simulink model "three_and_5_pole_jojo"  (R2025b)
settings: Solver=VariableStepAuto  StartTime=0.0  StopTime=20  RelTol=1e-3
model workspace (MAT data in the model file):
  Ki = 1546
  Kp = 7142.9
  Var = 0
  b = 50
  m = 1000
  u = 10
settings Model: Creator=clee1  LastModifiedBy=coven
settings SolverCC: AlgebraicLoopSolver=TrustRegion
settings DebuggingCC: UnconnectedInputMsg=warning  UnconnectedOutputMsg=warning  UnconnectedLineMsg=warning
settings ModelReferenceCC: EnableRefExpFcnMdlSchedulingChecks=on
settings RTWCC: GPUComputeCapability=3.5

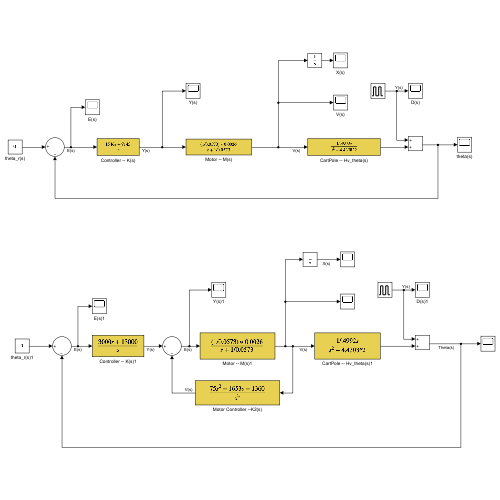
[thumbnail: Simulink's stored preview of the top-level diagram]
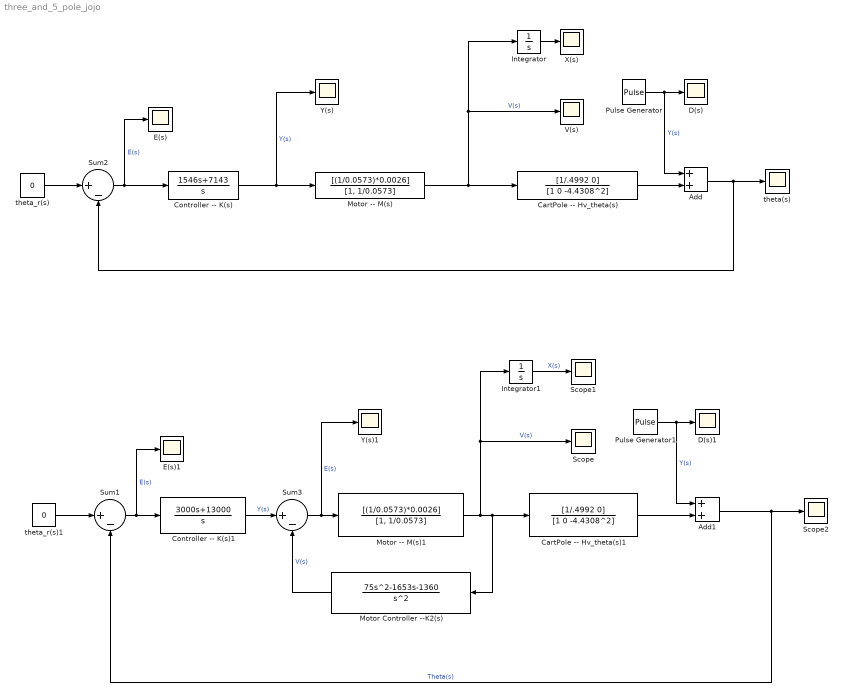
== system three_and_5_pole_jojo ==
  Add : Sum
  Add1 : Sum
  "CartPole -- Hv_theta(s)" : TransferFcn  Numerator=[1/.4992 0]  Denominator=[1 0 -4.4308^2]  ContinuousStateAttributes="\"Controller\""
  "CartPole -- Hv_theta(s)1" : TransferFcn  Numerator=[1/.4992 0]  Denominator=[1 0 -4.4308^2]  ContinuousStateAttributes="\"Controller\""
  "Controller -- K(s)" : TransferFcn  Numerator=[1546 7143]  Denominator=[1 0]  ContinuousStateAttributes="\"Controller\""
  "Controller -- K(s)1" : TransferFcn  Numerator=[3000 13000]  Denominator=[1 0]  ContinuousStateAttributes="\"Controller\""
  D(s) : Scope
      settings: ActiveDisplayYMinimum=-1  ActiveDisplayYMaximum=1  DataLoggingVariableName=ScopeData3
  D(s)1 : Scope
      settings: ActiveDisplayYMinimum=-0.018644180572280317  ActiveDisplayYMaximum=0.24786131822651522  DataLoggingVariableName=ScopeData6
  E(s) : Scope
      settings: ActiveDisplayYMinimum=-1  ActiveDisplayYMaximum=1  DataLoggingVariableName=ScopeData4
  E(s)1 : Scope
      settings: ActiveDisplayYMinimum=-1  ActiveDisplayYMaximum=1  DataLoggingVariableName=ScopeData7
  Integrator : Integrator
  Integrator1 : Integrator
  "Motor -- M(s)" : TransferFcn  Numerator=[(1/0.0573)*0.0026]  Denominator=[1, 1/0.0573]  ContinuousStateAttributes="\"Controller\""
  "Motor -- M(s)1" : TransferFcn  Numerator=[(1/0.0573)*0.0026]  Denominator=[1, 1/0.0573]  ContinuousStateAttributes="\"Controller\""
  Motor Controller --K2(s) : TransferFcn  Numerator=[75 -1653 -1360]  Denominator=[1 0 0 ]  ContinuousStateAttributes="\"Controller\""
  Pulse Generator : DiscretePulseGenerator  PulseType=Time based  Amplitude=0.3  Period=5
  Pulse Generator1 : DiscretePulseGenerator  PulseType=Time based  Amplitude=0.3  Period=5  PulseWidth=0.5
  Scope : Scope
      settings: ActiveDisplayYMinimum=-0.97614373938742749  ActiveDisplayYMaximum=0.53377649215921019  DataLoggingVariableName=ScopeData8
  Scope1 : Scope
      settings: ActiveDisplayYMinimum=-0.054339461276590076  ActiveDisplayYMaximum=0.09929346894755528  DataLoggingVariableName=ScopeData9
  Scope2 : Scope
      settings: ActiveDisplayYMinimum=-0.12997534985486678  ActiveDisplayYMaximum=0.34777503887276295  DataLoggingVariableName=ScopeData11
  Sum1 : Sum  Inputs=|+-
  Sum2 : Sum  Inputs=|+-
  Sum3 : Sum  Inputs=|+-
  V(s) : Scope
      settings: ActiveDisplayYMinimum=-1  ActiveDisplayYMaximum=1
  X(s) : Scope
      settings: ActiveDisplayYMinimum=-1  ActiveDisplayYMaximum=1  DataLoggingVariableName=ScopeData5
  Y(s) : Scope
      settings: ActiveDisplayYMinimum=-527.51671910279742  ActiveDisplayYMaximum=190.96907564842462  DataLoggingVariableName=ScopeData2
  Y(s)1 : Scope
      settings: ActiveDisplayYMinimum=-527.51671910279742  ActiveDisplayYMaximum=190.96907564842462  DataLoggingVariableName=ScopeData10
  theta(s) : Scope
      settings: ActiveDisplayYMinimum=-0.38730962768318911  ActiveDisplayYMaximum=0.46186138984333508
  theta_r(s) : Constant  Value=0
  theta_r(s)1 : Constant  Value=0
  wires:
  Sum2/1 -> E(s)/1, "Controller -- K(s)"/1  "E(s)"
  "Controller -- K(s)"/1 -> Y(s)/1, "Motor -- M(s)"/1  "Y(s)"
  "Motor -- M(s)"/1 -> "CartPole -- Hv_theta(s)"/1, V(s)/1, Integrator/1  "V(s)"
  "CartPole -- Hv_theta(s)"/1 -> Add/2
  Add/1 -> Sum2/2, theta(s)/1
  Pulse Generator/1 -> Add/1, D(s)/1  "Y(s)"
  theta_r(s)/1 -> Sum2/1
  Integrator/1 -> X(s)/1
  Add1/1 -> Scope2/1, Sum1/2  "Theta(s)"
  theta_r(s)1/1 -> Sum1/1
  Sum1/1 -> E(s)1/1, "Controller -- K(s)1"/1  "E(s)"
  "CartPole -- Hv_theta(s)1"/1 -> Add1/2
  "Motor -- M(s)1"/1 -> Motor Controller --K2(s)/1, "CartPole -- Hv_theta(s)1"/1, Scope/1, Integrator1/1  "V(s)"
  Pulse Generator1/1 -> Add1/1, D(s)1/1  "Y(s)"
  Integrator1/1 -> Scope1/1  "X(s)"
  "Controller -- K(s)1"/1 -> Sum3/1  "Y(s)"
  Sum3/1 -> Y(s)1/1, "Motor -- M(s)1"/1  "E(s)"
  Motor Controller --K2(s)/1 -> Sum3/2  "V(s)"
